simulink model "step3"  (R2021a)
settings: Solver=VariableStepAuto  StartTime=0.0  StopTime=10.0  RelTol=1e-3
settings Model: Creator=konsta  LastModifiedBy=konsta

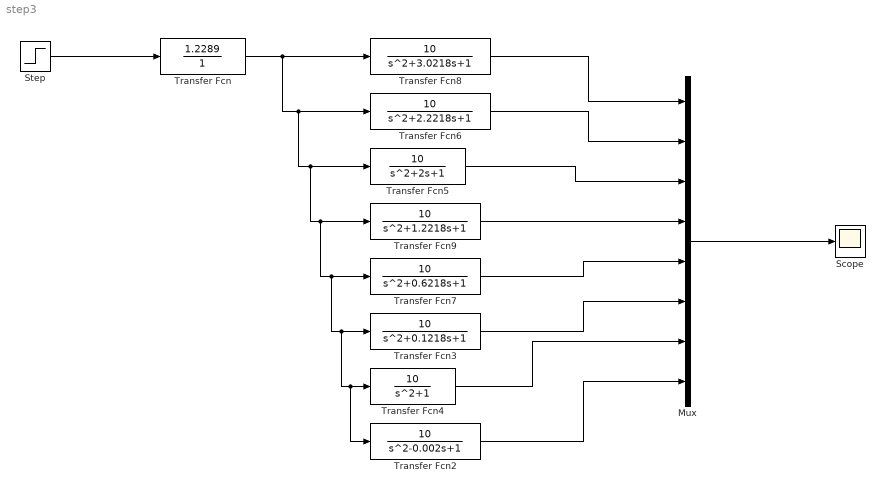
== system step3 ==
  Mux : Mux  Inputs=8
  Scope : Scope
  Step : Step  After=10*10^-6  SampleTime=0
  Transfer Fcn : TransferFcn  Numerator=[1.2289]  Denominator=[0 1]
  Transfer Fcn2 : TransferFcn  Numerator=[10]  Denominator=[1 -0.002 1]
  Transfer Fcn3 : TransferFcn  Numerator=[10]  Denominator=[1 0.1218 1]
  Transfer Fcn4 : TransferFcn  Numerator=[10]  Denominator="[1 0  1]"
  Transfer Fcn5 : TransferFcn  Numerator=[10]
  Transfer Fcn6 : TransferFcn  Numerator=[10]  Denominator=[1 2.2218 1]
  Transfer Fcn7 : TransferFcn  Numerator=[10]  Denominator=[1 0.6218 1]
  Transfer Fcn8 : TransferFcn  Numerator=[10]  Denominator=[1 3.0218 1]
  Transfer Fcn9 : TransferFcn  Numerator=[10]  Denominator=[1 1.2218 1]
  wires:
  Transfer Fcn/1 -> Transfer Fcn2/1, Transfer Fcn4/1, Transfer Fcn3/1, Transfer Fcn7/1, Transfer Fcn9/1, Transfer Fcn5/1, Transfer Fcn6/1, Transfer Fcn8/1
  Mux/1 -> Scope/1
  Transfer Fcn8/1 -> Mux/1
  Transfer Fcn2/1 -> Mux/8
  Transfer Fcn4/1 -> Mux/7
  Transfer Fcn3/1 -> Mux/6
  Transfer Fcn7/1 -> Mux/5
  Transfer Fcn9/1 -> Mux/4
  Transfer Fcn5/1 -> Mux/3
  Transfer Fcn6/1 -> Mux/2
  Step/1 -> Transfer Fcn/1
